simulink model "dyn_compononents_test"  (R2025b)
settings: Solver=ode1  StartTime=0.0  StopTime=20  FixedStep=dt  RelTol=1e-3
model workspace (MAT data in the model file):
  dt = 0.001
libraries: sdu_controllers x5
settings Model: Creator=eld  LastModifiedBy=madla

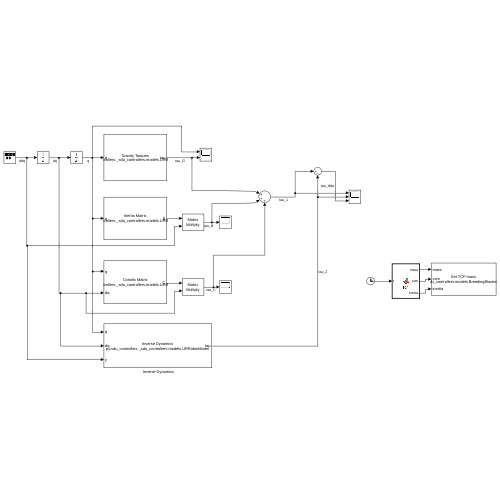
[thumbnail: Simulink's stored preview of the top-level diagram]
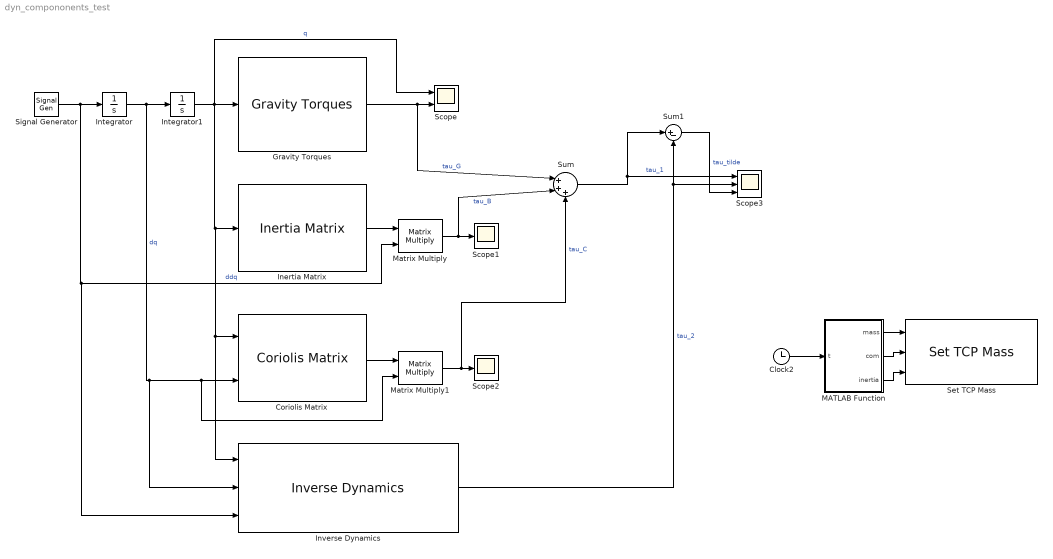
== system dyn_compononents_test ==
  " Inverse Dynamics" : sdu_controllers/Dynamics/Inverse Dynamics  robot_model=ur3e  SimulateUsing=Interpreted execution
      settings: SourceProductName=SDU Controllers
  Clock2 : Clock
  Coriolis Matrix : sdu_controllers/Dynamics/Coriolis Matrix  robot_model=ur3e  SimulateUsing=Interpreted execution
      settings: SourceProductName=SDU Controllers
  Gravity Torques : sdu_controllers/Dynamics/Gravity Torques  robot_model=ur3e  SimulateUsing=Interpreted execution
      settings: SourceProductName=SDU Controllers
  Inertia Matrix : sdu_controllers/Dynamics/Inertia Matrix  robot_model=ur3e  SimulateUsing=Interpreted execution
      settings: SourceProductName=SDU Controllers
  Integrator : Integrator
  Integrator1 : Integrator
  MATLAB Function : MATLAB Function  TreatAsAtomicUnit=on
  Matrix Multiply : Product  Multiplication=Matrix(*)
  Matrix Multiply1 : Product  Multiplication=Matrix(*)
  Scope : Scope  NumInputPorts=2
      settings: ActiveDisplayYMinimum=-0.9549392571864036  ActiveDisplayYMaximum=8.5944533146776347
  Scope1 : Scope
      settings: ActiveDisplayYMinimum=-1.24045  ActiveDisplayYMaximum=1.25732
  Scope2 : Scope
      settings: ActiveDisplayYMinimum=-0.55947  ActiveDisplayYMaximum=0.25783  DataLoggingVariableName=ScopeData2
  Scope3 : Scope  NumInputPorts=3
      settings: ActiveDisplayYMinimum=-85.769130530019481  ActiveDisplayYMaximum=51.058170971414093  DataLoggingVariableName=ScopeData3
  Set TCP Mass : sdu_controllers/Dynamics/Set TCP Mass  robot_model=bbrobot  SimulateUsing=Interpreted execution
      settings: SourceProductName=SDU Controllers
  Signal Generator : SignalGenerator  Amplitude=ones(6,1)  Frequency=ones(6,1)+pi/2  Units=rad/sec
  Sum : Sum  Inputs=|+++
  Sum1 : Sum  Inputs=|+-
  wires:
  Integrator1/1 -> Gravity Torques/1, " Inverse Dynamics"/1, Coriolis Matrix/1, Inertia Matrix/1, Scope/1  "q"
  Integrator/1 -> " Inverse Dynamics"/2, Matrix Multiply1/2, Coriolis Matrix/2, Integrator1/1  "dq"
  Signal Generator/1 -> " Inverse Dynamics"/3, Matrix Multiply/2, Integrator/1  "ddq"
  Gravity Torques/1 -> Sum/1, Scope/2  "tau_G"
  Inertia Matrix/1 -> Matrix Multiply/1
  Matrix Multiply/1 -> Sum/2, Scope1/1  "tau_B"
  Coriolis Matrix/1 -> Matrix Multiply1/1
  Matrix Multiply1/1 -> Sum/3, Scope2/1  "tau_C"
  Sum/1 -> Sum1/1, Scope3/1  "tau_1"
  " Inverse Dynamics"/1 -> Sum1/2, Scope3/2  "tau_2"
  Sum1/1 -> Scope3/3  "tau_tilde"
  MATLAB Function/2(com) -> Set TCP Mass/2
  MATLAB Function/3(inertia) -> Set TCP Mass/3
  Clock2/1 -> MATLAB Function/1(t)
  MATLAB Function/1(mass) -> Set TCP Mass/1

== matlab function dyn_compononents_test/MATLAB Function ==
  data: t input; mass output; com output; inertia output
function [mass, com, inertia] = fcn(t)

if t < 10
    mass = 0;
    com = [0 0 0];
    inertia = zeros(3, 3);
else
    mass = 1;
    com = [0 0 0.2];
    inertia = 1 * eye(3);
end
